simulink model "boucleferm"  (R2013a)
settings: Solver=ode45  StartTime=0.0  StopTime=20  RelTol=1e-3
undefined symbols (not defined in the file): A, B, C, D, fdesignblkfcn, gcbh
libraries: simulink x4
settings Model: Creator=user  LastModifiedBy=user
settings OptimizationCC: OptimizeModelRefInitCode=on  LifeSpan=1
settings DebuggingCC: StrictBusMsg=Warning
settings HardwareCC: ProdBitPerInt=16  ProdBitPerPointer=8  ProdIntDivRoundTo=Zero  ProdEndianess=LittleEndian  ProdWordSize=8  ProdHWDeviceType=Atmel->AVR
settings RTWCC: SystemTargetFile=realtime.tlc  GenerateMakefile=off  TemplateMakefile=realtime.tmf  Description=Run on Target Hardware  RTWVerbose=off  ProcessScript=realtime_make_rtw_hook
settings CodeAppCC: IgnoreCustomStorageClasses=off
settings STFCustomTargetCC: TargetLibSuffix=.a  GenerateSampleERTMain=on  CombineOutputUpdateFcns=on  ERTCustomFileBanners=on  SupportContinuousTime=off  SupportNonInlinedSFcns=off  MATLABClassNameForMDSCustomization=Simulink.SoftwareTarget.ERTCustomization  SystemTargetFile=realtime.tlc
settings ERTTargetCC: ParMdlRefBuildCompliant=off  CompOptLevelCompliant=off  ConcurrentExecutionCompliant=off  ERTFirstTimeCompliant=off  ModelStepFunctionPrototypeControlCompliant=off  CPPClassGenCompliant=off  ERTCustomFileTemplate=realtime_file_process.tlc

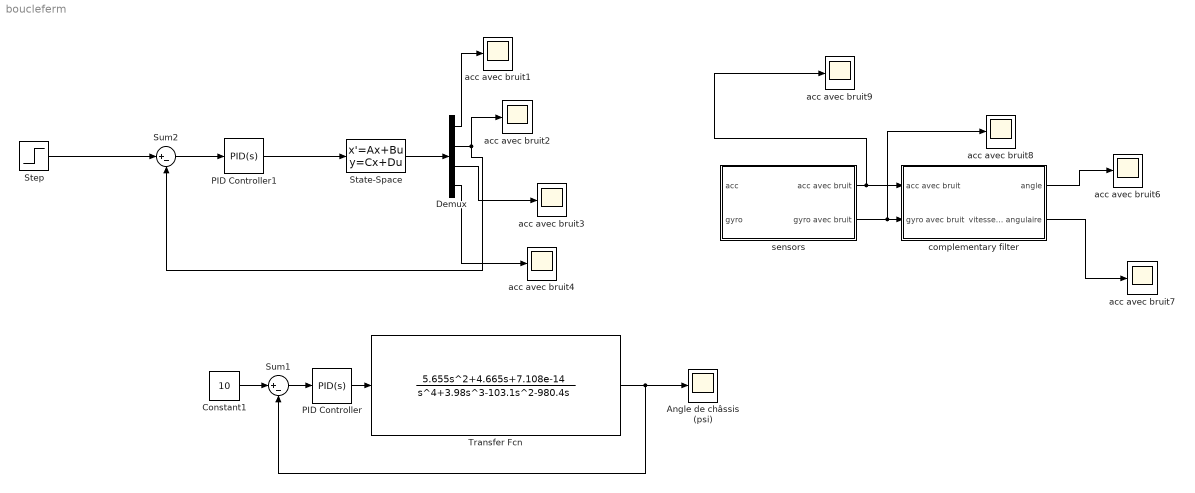
== system boucleferm ==
  "Angle de châssis (psi) " : Scope
      settings: TimeRange=10  YMin=-175.044  YMax=-175.043  SaveName=ScopeData7
  Constant1 : Constant  Value=10
  Demux : Demux
  PID Controller : simulink/Continuous/PID Controller  Controller=PID  TimeDomain=Continuous-time  SampleTime=1  IntegratorMethod=Forward Euler  FilterMethod=Forward Euler  Form=Parallel  P=134.990450216863  I=388.273311298141  D=5.07878900537804  N=35.0391468351183  InitialConditionSource=internal  InitialConditionForIntegrator=0  InitialConditionForFilter=0  ExternalReset=none  LimitOutput=off  UpperSaturationLimit=inf  LowerSaturationLimit=-inf  LinearizeAsGain=on  AntiWindupMode=none  Kb=1  TrackingMode=off  Kt=1  PParamMin=[]  PParamMax=[]  IParamMin=[]  IParamMax=[]  DParamMin=[]  DParamMax=[]  NParamMin=[]  NParamMax=[]  KbParamMin=[]  KbParamMax=[]  KtParamMin=[]  KtParamMax=[]  POutMin=[]  POutMax=[]  IOutMin=[]  IOutMax=[]  DOutMin=[]  DOutMax=[]  NOutMin=[]  NOutMax=[]  KbOutMin=[]  KbOutMax=[]  KtOutMin=[]  KtOutMax=[]  IntegratorOutMin=[]  IntegratorOutMax=[]  FilterOutMin=[]  FilterOutMax=[]  SumOutMin=[]  SumOutMax=[]  SumI1OutMin=[]  SumI1OutMax=[]  SumI2OutMin=[]  SumI2OutMax=[]  SumI3OutMin=[]  SumI3OutMax=[]  SumDOutMin=[]  SumDOutMax=[]  SaturationOutMin=[]  SaturationOutMax=[]  IntegratorContinuousStateAttributes=''  IntegratorStateMustResolveToSignalObject=off  IntegratorRTWStateStorageClass=Auto  FilterContinuousStateAttributes=''  FilterStateMustResolveToSignalObject=off  FilterRTWStateStorageClass=Auto
  PID Controller1 : simulink/Continuous/PID Controller  Controller=PID  TimeDomain=Continuous-time  SampleTime=1  IntegratorMethod=Forward Euler  FilterMethod=Forward Euler  Form=Parallel  P=654.195498547375  I=957.521144572743  D=33.9395149282384  N=387.31370109608  InitialConditionSource=internal  InitialConditionForIntegrator=0  InitialConditionForFilter=0  ExternalReset=none  LimitOutput=off  UpperSaturationLimit=inf  LowerSaturationLimit=-inf  LinearizeAsGain=on  AntiWindupMode=none  Kb=1  TrackingMode=off  Kt=1  PParamMin=[]  PParamMax=[]  IParamMin=[]  IParamMax=[]  DParamMin=[]  DParamMax=[]  NParamMin=[]  NParamMax=[]  KbParamMin=[]  KbParamMax=[]  KtParamMin=[]  KtParamMax=[]  POutMin=[]  POutMax=[]  IOutMin=[]  IOutMax=[]  DOutMin=[]  DOutMax=[]  NOutMin=[]  NOutMax=[]  KbOutMin=[]  KbOutMax=[]  KtOutMin=[]  KtOutMax=[]  IntegratorOutMin=[]  IntegratorOutMax=[]  FilterOutMin=[]  FilterOutMax=[]  SumOutMin=[]  SumOutMax=[]  SumI1OutMin=[]  SumI1OutMax=[]  SumI2OutMin=[]  SumI2OutMax=[]  SumI3OutMin=[]  SumI3OutMax=[]  SumDOutMin=[]  SumDOutMax=[]  SaturationOutMin=[]  SaturationOutMax=[]  IntegratorContinuousStateAttributes=''  IntegratorStateMustResolveToSignalObject=off  IntegratorRTWStateStorageClass=Auto  FilterContinuousStateAttributes=''  FilterStateMustResolveToSignalObject=off  FilterRTWStateStorageClass=Auto
  State-Space : StateSpace  A=A  B=B  C=C  D=D
  Step : Step  Before=1  SampleTime=0
  Sum1 : Sum  Inputs=|+-
  Sum2 : Sum  Inputs=|+-
  Transfer Fcn : TransferFcn  Numerator=[5.655 4.665 7.108e-14]  Denominator=[1 3.98 -103.1 -980.4 0]
  acc avec bruit{1..4,6..9} (8 alike) : Scope
      acc avec bruit1 settings: TimeRange=10  YMin=-175.044  YMax=-175.043  SaveName=ScopeData3
      acc avec bruit2 settings: TimeRange=20  YMin=0  YMax=12  SaveName=ScopeData4
      acc avec bruit3 settings: TimeRange=10  YMin=-175.044  YMax=-175.043  SaveName=ScopeData5
      acc avec bruit4 settings: TimeRange=10  YMin=-175.044  YMax=-175.043  SaveName=ScopeData6
      acc avec bruit6 settings: TimeRange=20  YMin=-1.2e+99  YMax=1.999999999999999e+98
      acc avec bruit7 settings: TimeRange=10  YMin=-175.044  YMax=-175.043
      acc avec bruit8 settings: TimeRange=20  YMin=-1.2e+99  YMax=1.999999999999999e+98  SaveName=ScopeData2
      acc avec bruit9 settings: TimeRange=20  YMin=-1.2e+99  YMax=1.999999999999999e+98  SaveName=ScopeData8
  complementary filter : Subsystem
  sensors : Subsystem
  wires:
  State-Space/1 -> Demux/1
  Demux/3 -> acc avec bruit3/1
  Demux/4 -> acc avec bruit4/1
  Demux/1 -> acc avec bruit1/1
  Transfer Fcn/1 -> Sum1/2, "Angle de châssis (psi) "/1
  Constant1/1 -> Sum1/1
  PID Controller/1 -> Transfer Fcn/1
  Sum1/1 -> PID Controller/1
  Sum2/1 -> PID Controller1/1
  Demux/2 -> acc avec bruit2/1, Sum2/2
  sensors/2("gyro avec bruit  ") -> acc avec bruit8/1, complementary filter/2("gyro avec bruit ")
  complementary filter/1("angle ") -> acc avec bruit6/1
  complementary filter/2(vitesse angulaire) -> acc avec bruit7/1
  PID Controller1/1 -> State-Space/1
  Step/1 -> Sum2/1
  sensors/1("acc avec bruit ") -> acc avec bruit9/1, complementary filter/1("acc avec bruit ")

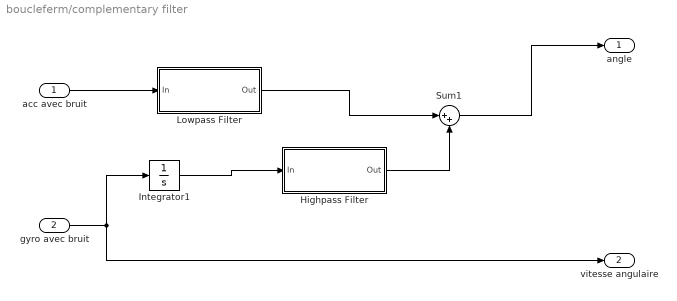
== system boucleferm/complementary filter ==
  "acc avec bruit " : Inport
  "gyro avec bruit " : Inport  Port=2
  Highpass Filter : Subsystem  DialogController=fdesignblkfcn  InitFcn=fdesignblkfcn(gcbh, {'InitFcn'});  mask(Highpass Filter){}
      mask help: Design a highpass filter
      settings: CopyFcn=fdesignblkfcn(gcbh, {'CopyFcn'});
      mask Help: helpview(mapfilelocation('dsp'), 'dsphighpassfilter');
      mask Display: disp('Highpass')
  Integrator1 : Integrator  InitialCondition=1
  Lowpass Filter : Subsystem  DialogController=fdesignblkfcn  InitFcn=fdesignblkfcn(gcbh, {'InitFcn'});  mask(Lowpass Filter){}
      mask help: Design a lowpass filter
      settings: CopyFcn=fdesignblkfcn(gcbh, {'CopyFcn'});
      mask Help: helpview(mapfilelocation('dsp'), 'dsplowpassfilter');
      mask Display: disp('Lowpass')
  Sum1 : Sum  Inputs=|++
  "angle " : Outport
  vitesse angulaire : Outport  Port=2
  wires:
  Sum1/1 -> "angle "/1
  "acc avec bruit "/1 -> Lowpass Filter/1(In)
  "gyro avec bruit "/1 -> Integrator1/1, vitesse angulaire/1
  Integrator1/1 -> Highpass Filter/1(In)
  Highpass Filter/1(Out) -> Sum1/2
  Lowpass Filter/1(Out) -> Sum1/1

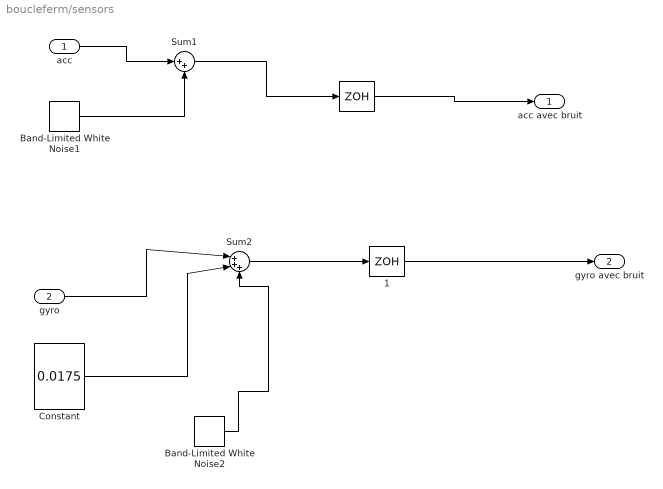
== system boucleferm/sensors ==
  acc : Inport
  gyro : Inport  Port=2
  " " : ZeroOrderHold
  " 1" : ZeroOrderHold
  Band-Limited White Noise1 : simulink/Sources/Band-Limited White Noise  Cov=[0.9]  Ts=0.1  seed=[23341]
  Band-Limited White Noise2 : simulink/Sources/Band-Limited White Noise  Cov=[0.9]  Ts=0.1  seed=[23341]
  Constant : Constant  Value=0.0175
  Sum1 : Sum  Inputs=|++
  Sum2 : Sum  Inputs=|+++
  "acc avec bruit " : Outport
  "gyro avec bruit  " : Outport  Port=2
  wires:
  acc/1 -> Sum1/1
  Band-Limited White Noise1/1 -> Sum1/2
  Constant/1 -> Sum2/2
  Sum1/1 -> " "/1
  " "/1 -> "acc avec bruit "/1
  gyro/1 -> Sum2/1
  Sum2/1 -> " 1"/1
  Band-Limited White Noise2/1 -> Sum2/3
  " 1"/1 -> "gyro avec bruit  "/1

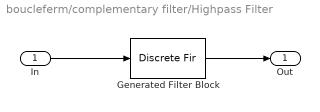
== system boucleferm/complementary filter/Highpass Filter ==
  In : Inport
  Generated Filter Block : DiscreteFir  Tag=BlockMethodSubSystem  Coefficients=[-0.001713682665110306 0.0083143784480805769 -0.012717355233486931 0.0055609517902503753 0.0073397102425536197 -0.006531049050179258 -0.0076900499697794954 0.0090269831680985079 0.0088388618995090904 -0.012960741353766195 -0.010074958667252783 0.018520174010008873 0.011233354613588929 -0.026375248383613631 -0.012270782185765867 0.038180976692389727 0.013130425918293593 -0.058293359325192265 -0.013768295948648092 0.102813257992074 0.014167876773854067 -0.31720255241603534 0.48569804617051759 -0.31720255241603534 0.014167876773854067 0.102813257992074 -0.013768295948648092 -0.058293359325192265 0.013130425918293593 0.038180976692389727 -0.012270782185765867 -0.026375248383613631 0.011233354613588929 0.018520174010008873 -0.010074958667252783 -0.012960741353766195 0.0088388618995090904 0.0090269831680985079 -0.0076900499697794954 -0.006531049050179258 0.0073397102425536197 0.0055609517902503753 -0.012717355233486931 0.0083143784480805769 -0.001713682665110306]  InputProcessing=Columns as channels (frame based)
  Out : Outport
  wires:
  Generated Filter Block/1 -> Out/1
  In/1 -> Generated Filter Block/1

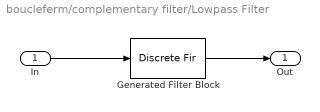
== system boucleferm/complementary filter/Lowpass Filter ==
  In : Inport
  Generated Filter Block : DiscreteFir  Tag=BlockMethodSubSystem  Coefficients=[-0.0024228738523269142 -0.002083244982079274 0.0067703446401187091 0.016731945423489058 0.011117076081077608 -0.0062311454141445394 -0.008401617186026911 0.0092567976151380175 0.012982883808855752 -0.010121234703278968 -0.018273518733782485 0.011431962071777957 0.02617588858040763 -0.012489027835322923 -0.037996623145463579 0.013388945199366963 0.058155465814729891 -0.014048043515808939 -0.10272466857882172 0.014462275771238358 0.31716649721769491 0.48538764678732504 0.31716649721769491 0.014462275771238358 -0.10272466857882172 -0.014048043515808939 0.058155465814729891 0.013388945199366963 -0.037996623145463579 -0.012489027835322923 0.02617588858040763 0.011431962071777957 -0.018273518733782485 -0.010121234703278968 0.012982883808855752 0.0092567976151380175 -0.008401617186026911 -0.0062311454141445394 0.011117076081077608 0.016731945423489058 0.0067703446401187091 -0.002083244982079274 -0.0024228738523269142]  InputProcessing=Columns as channels (frame based)
  Out : Outport
  wires:
  In/1 -> Generated Filter Block/1
  Generated Filter Block/1 -> Out/1
